simulink library "euler"  (R2020b)
settings: Solver=VariableStepAuto  StartTime=0.0  StopTime=10.0  RelTol=1e-3
values from neighbouring files (symbols this model uses):
  phi0 = 0.0    (= 0)    [initial_conditions.m]
  psi0 = 0.0    (= 0)    [initial_conditions.m]
  theta0 = 1    [initial_conditions.m]
settings Model: Creator=whitehole  LastModifiedBy=whitehole

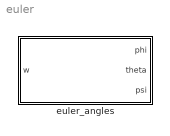
== system euler ==
  euler_angles : Subsystem

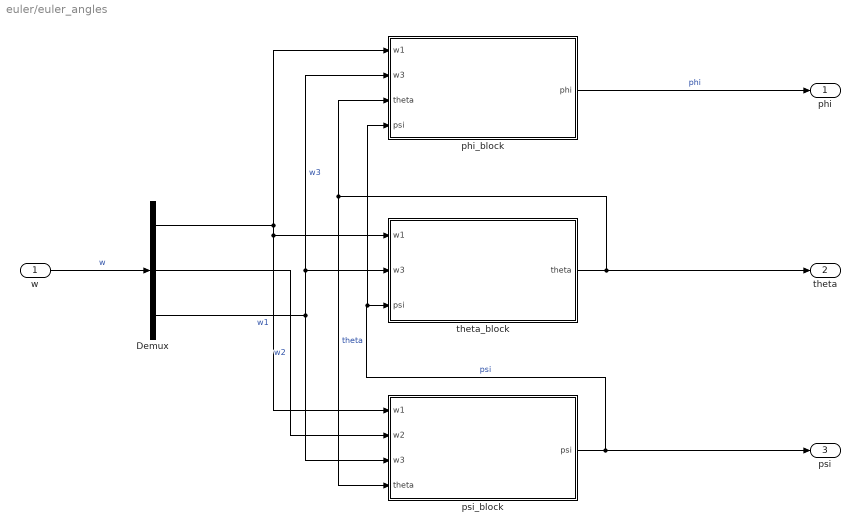
== system euler/euler_angles ==
  w : Inport
  Demux : Demux  Outputs=3
  phi_block : Subsystem
  psi_block : Subsystem
  theta_block : Subsystem
  phi : Outport
  theta : Outport  Port=2
  psi : Outport  Port=3
  wires:
  w/1 -> Demux/1  "w"
  phi_block/1(phi) -> phi/1  "phi"
  psi_block/1(psi) -> phi_block/4(psi), theta_block/3(psi), psi/1  "psi"
  theta_block/1(theta) -> phi_block/3(theta), psi_block/4(theta), theta/1  "theta"
  Demux/1 -> psi_block/1(w1), theta_block/1(w1), phi_block/1(w1)  "w1"
  Demux/3 -> theta_block/2(w3), phi_block/2(w3), psi_block/3(w3)  "w3"
  Demux/2 -> psi_block/2(w2)  "w2"

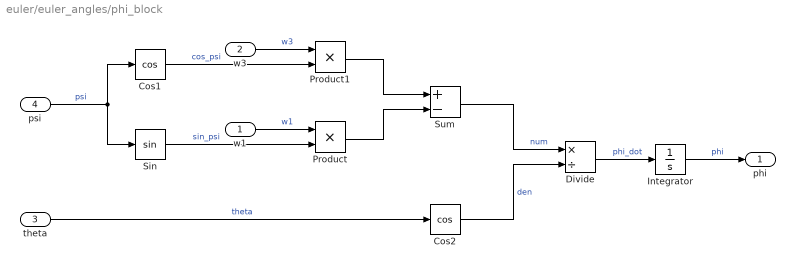
== system euler/euler_angles/phi_block ==
  w1 : Inport
  w3 : Inport  Port=2
  theta : Inport  Port=3
  psi : Inport  Port=4
  Cos1 : Trigonometry  Operator=cos
  Cos2 : Trigonometry  Operator=cos
  Divide : Product  Inputs=*/
  Integrator : Integrator  InitialCondition=phi0  WrapState=on
  Product : Product
  Product1 : Product
  Sin : Trigonometry
  Sum : Sum  Inputs=+-
  phi : Outport
  wires:
  theta/1 -> Cos2/1  "theta"
  psi/1 -> Sin/1, Cos1/1  "psi"
  Divide/1 -> Integrator/1  "phi_dot"
  w1/1 -> Product/1  "w1"
  w3/1 -> Product1/1  "w3"
  Sin/1 -> Product/2  "sin_psi"
  Cos1/1 -> Product1/2  "cos_psi"
  Product/1 -> Sum/2
  Product1/1 -> Sum/1
  Sum/1 -> Divide/1  "num"
  Cos2/1 -> Divide/2  "den"
  Integrator/1 -> phi/1  "phi"

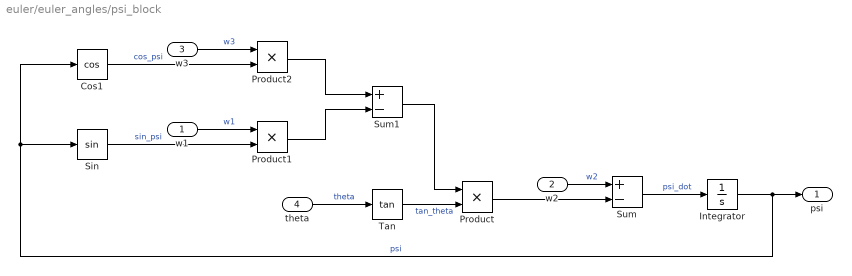
== system euler/euler_angles/psi_block ==
  w1 : Inport
  w2 : Inport  Port=2
  w3 : Inport  Port=3
  theta : Inport  Port=4
  Cos1 : Trigonometry  Operator=cos
  Integrator : Integrator  InitialCondition=psi0  WrapState=on
  Product : Product
  Product1 : Product
  Product2 : Product
  Sin : Trigonometry
  Sum : Sum  Inputs=+-
  Sum1 : Sum  Inputs=+-
  Tan : Trigonometry  Operator=tan
  psi : Outport
  wires:
  Integrator/1 -> Sin/1, Cos1/1, psi/1  "psi"
  Sum/1 -> Integrator/1  "psi_dot"
  w2/1 -> Sum/1  "w2"
  theta/1 -> Tan/1  "theta"
  Tan/1 -> Product/2  "tan_theta"
  Sin/1 -> Product1/2  "sin_psi"
  w1/1 -> Product1/1  "w1"
  w3/1 -> Product2/1  "w3"
  Product2/1 -> Sum1/1
  Product1/1 -> Sum1/2
  Cos1/1 -> Product2/2  "cos_psi"
  Product/1 -> Sum/2
  Sum1/1 -> Product/1

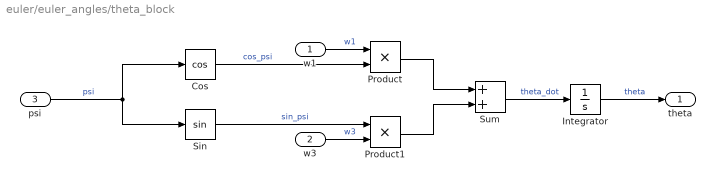
== system euler/euler_angles/theta_block ==
  w1 : Inport
  w3 : Inport  Port=2
  psi : Inport  Port=3
  Cos : Trigonometry  Operator=cos
  Integrator : Integrator  InitialCondition=theta0  WrapState=on
  Product : Product
  Product1 : Product
  Sin : Trigonometry
  Sum : Sum
  theta : Outport
  wires:
  Cos/1 -> Product/2  "cos_psi"
  Sin/1 -> Product1/1  "sin_psi"
  psi/1 -> Cos/1, Sin/1  "psi"
  w1/1 -> Product/1  "w1"
  w3/1 -> Product1/2  "w3"
  Product/1 -> Sum/1
  Product1/1 -> Sum/2
  Sum/1 -> Integrator/1  "theta_dot"
  Integrator/1 -> theta/1  "theta"
